simulink library "AVE_Library"  (R2025b)
settings: Solver=VariableStepAuto  StartTime=0.0  StopTime=10.0  RelTol=1e-3
undefined symbols (not defined in the file or in its folder): DiscIntNeverNeededParam
libraries: simulink x44, etargetslib x18, $bdroot x13, GenericTarget x2
(part 1 of 5)
settings Model: Creator=Scythe  LastModifiedBy=damerius
settings SolverCC: AlgebraicLoopSolver=TrustRegion
settings DataIOCC: ReturnWorkspaceOutputs=off
settings OptimizationCC: ReuseModelBlockBuffer=off
settings DebuggingCC: UnconnectedInputMsg=warning  UnconnectedOutputMsg=warning  UnconnectedLineMsg=warning  ArithmeticOperatorsInVariantConditions=warning
settings ModelReferenceCC: EnableRefExpFcnMdlSchedulingChecks=on
settings SFSimCC: CustomCodeUndefinedFunction=UseInterfaceOnly
settings RTWCC: GPUComputeCapability=3.5  DLArmComputeVersion=19.05

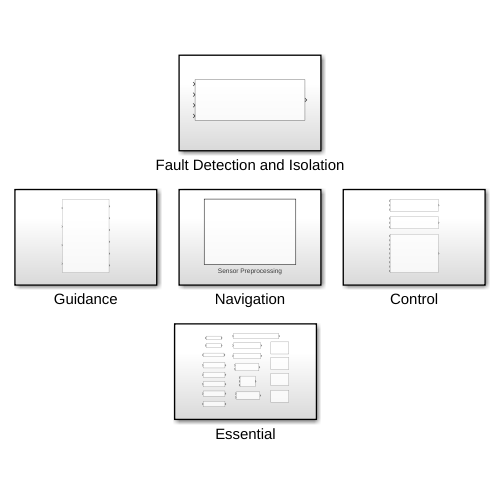
[thumbnail: Simulink's stored preview of the top-level diagram]
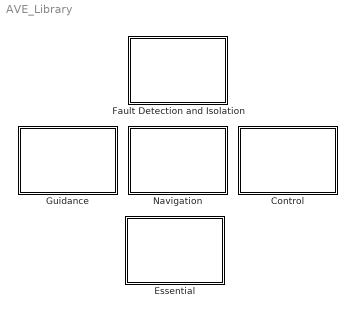
== system AVE_Library ==
  Control : Subsystem
  Essential : Subsystem
  Fault Detection and Isolation : Subsystem
  Guidance : Subsystem
  Navigation : Subsystem

== system AVE_Library/Control ==
  Aperiodic IT2 SISO Control with Integral Action and Input Delay : Subsystem  mask{maxNumDelays=20, SampleTime=0.01}
      mask prompts: maxNumDelays "Max. number of delays:"; SampleTime "Sample time:"
      mask help:
      | Aperiodic SISO controller with integral action for an IT2 process with input delay. The controller is designed online when parameters are changed. The input <b>gamma</b> sets the performance of the controller (<i>mu</i> and <i>beta</i> are optional tuning parameters and can be left to their default values).<br><br>
      | The state-space model being controlled is given by:<br>
      | A = [0 1 0; 0 -1/T1 k/T1; 0 0 -1/T2]<br>
      | B = [0; 0; 1/T2]<br>
      | C = [1 0 0]<br>
      | <br><br>
      | To compensate for input delays, this block stores the previous input values in a ring buffer. The maximum size of the ring buffer is set via the block mask parameter below.
      | <br><br>
      | <table border="1" align="center" width="100%"><tr><th>Input</th></tr></table><br><br>
      | <b>yr_minus_y</b><br>
      | The control error given by the difference of reference value <i>yr</i> and output value <i>y</i>.<br><br>
      | <b>x</b><br>
      | The three-dimensional state vector.<br><br>
      | <table border="1" align="center" width="100%"><tr><th>Input / Parameter</th></tr></table><br><br>
      | <b>k</b>, <b>T1</b>, <b>T2</b><br>Gain and timeconstants of the IT2 process.<br><br>
      | <b>gamma</b> (0,inf)<br>Performance parameter for control design: dominant eigenvalue of closed loop system should be gamma times dominant eigenvalue of model (1/max(T1,T2)). Greater values result in higher performance.<br><br>
      | <b>mu</b> [1, inf)<br>Default value: 2. Spreads 4 poles of closed loop system to the left based on dominant closed loop eigenvalue. A value of 1 means: all poles of closed loop system should be equal to the dominant pole.<br><br>
      | <b>beta</b> [0, inf)<br>Default value: 1. Adjusts the anti-windup gain for back calculation. A value of zero disables back calculation.<br><br>
      | <b>inputTimeDelay</b> [0,inf)<br>Input delay of the process in seconds or zero if the process has no input delay. Internally, this value is rounded to multiples of the sample time and is also clamped to the maximum possible input delay depending on the input ring buffer size.<br><br>
      | <b>saturationLimits</b><br>A two-dimensional vector containing the lower and upper saturation limits. The order does not matter: internally the greatest and lowest value of both are used as upper and lower limit, respectively.<br><br>
      | <b>reset</b><br>Reset the controller by forcing all storage values to zero, including integrator state and the ring buffer for delayed inputs.<br><br>
      | <table border="1" align="center" width="100%"><tr><th>Output</th></tr></table><br><br>
      | <b>u</b><br>The saturated control input to be applied to the process.
      mask DialogControl DescGroupVar Prompt: Aperiodic IT2 SISO Control with Integral Action and Input Delay
      mask Display: disp('Aperiodic IT2 SISO Control\n(Integral Action)\n(Input Delay)');
  Input Delay Compensation : Subsystem  mask{dimU=1, dimX=2, maxNumDelays=20, SampleTime=0.01}
      mask prompts: dimU "Input dimension:"; dimX "State dimension:"; maxNumDelays "Max. number of delays:"; SampleTime "Sample time:"
      mask help:
      | Calculate the input delay compensation term based on the input value of the previous time step and the designed compensation weights. Use this block in conjunction with the "Input Delay Compensation Design" block.<br>
      | This block stores all input values u_prev in a ring buffer and weights all of them by the delayWeights to calculate the compensation term xc. Use the reset input to reset the buffer to zero before storing the input value.<br>
      | <br>
      | <b>Details</b><br>
      | To consider input delays for a linear state space [<i><b>A</b></i>, <i><b>B</b></i>] with control law <i><b>u</b> = -<b>K</b>*<b>x</b></i>, the control law should be replaced by <i><b>u</b> = -<b>Kc</b> * (<b>x</b> + <b>xc</b>)</i>, where <i><b>Kc</b></i> is designed for the state space [<i><b>A</b></i>, <i>expm(-<b>A</b>*h)*<b>B</b></i>] and <i>h &gt; 0</i> is the input delay. <i><b>xc</b></i> is denoted as the compensation term given by the integral of <i>expm(-<b>A</b>*(s+h))*<b>B</b>*u(t+s)</i> over the time interval <i>s=[-h, 0]</i>. For more details, view the reference.
      | <br>
      | <br>
      | <i>Reference<br>
      | Kwon, W. and Pearson, A. (1980). Feedback stabilization of linear systems with delayed control. IEEE Transactions on Automatic Control, 25(2), 266–269. doi:10.1109/TAC.1980.1102288.</i>
      mask DialogControl DescGroupVar Prompt: Input Delay Compensation
      mask Display: disp('Input Delay Compensation');
  Input Delay Compensation Design : Subsystem  mask{dimU=1, dimX=2, maxNumDelays=20, SampleTime=0.01}
      mask prompts: dimU "Input dimension:"; dimX "State dimension:"; maxNumDelays "Max. number of delays:"; SampleTime "Sample time (for design only):"
      mask help:
      | Design weighting matrix for an input delay compensation system. Use this block in conjunction with an "Input Delay Compensation" block. inputDelaySteps represent the input delay in number of discrete time steps with a sampletime specified via the block mask. The sample time parameter is only used to calculate the delay weights. It does not affect the execution of this block.<br>
      | <br>
      | <b>Details</b><br>
      | To consider input delays for a linear state space [<i><b>A</b></i>, <i><b>B</b></i>] with control law <i><b>u</b> = -<b>K</b>*<b>x</b></i>, the control law should be replaced by <i><b>u</b> = -<b>Kc</b> * (<b>x</b> + <b>xc</b>)</i>, where <i><b>Kc</b></i> is designed for the state space [<i><b>A</b></i>, <i>expm(-<b>A</b>*h)*<b>B</b></i>] and <i>h &gt; 0</i> is the input delay. <i><b>xc</b></i> is denoted as the compensation term given by the integral of <i>expm(-<b>A</b>*(s+h))*<b>B</b>*u(t+s)</i> over the time interval <i>s=[-h, 0]</i>. For more details, view the reference.
      | <br>
      | <br>
      | <i>Reference<br>
      | Kwon, W. and Pearson, A. (1980). Feedback stabilization of linear systems with delayed control. IEEE Transactions on Automatic Control, 25(2), 266–269. doi:10.1109/TAC.1980.1102288.</i>
      mask DialogControl DescGroupVar Prompt: Input Delay Compensation Design
      mask Display: disp('Input Delay Compensation\nDesign');

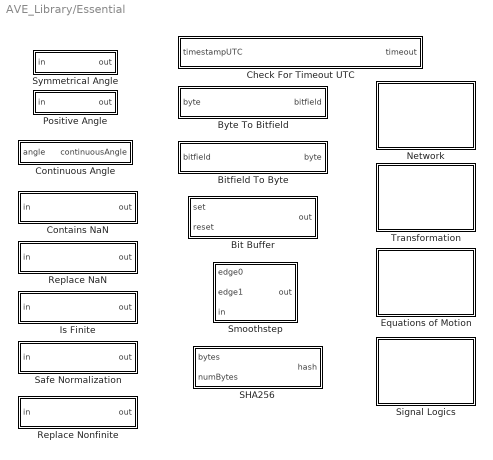
== system AVE_Library/Essential ==
  Bit Buffer : Subsystem  mask{dataType=uint8}
      mask prompts: dataType "Data type:"
      mask help: This block stores all bits in a buffer. All bits from the input "set" are set using bitwise OR of input and buffer. All bits in the buffer remain high until the corresponding bit is reset using the "reset" input. "reset" always overwrites "set".
      mask DialogControl DescGroupVar Prompt: Bit Buffer
      mask Display:
      | type = get_param(gcb, 'dataType');
      | disp(['Bit Buffer\n(' type ')']);
  Bitfield To Byte : Subsystem
      mask help: Convert a bitfield of 8 bits to a single byte. The input bitfield must be a vector containing 8 boolean values where the first value indicates whether the LSBit is to be set or not.
      mask DialogControl DescGroupVar Prompt: Bitfield To Byte
      mask Display: text(0.5, 0.5, 'Bitfield to Byte', 'horizontalAlignment', 'center');
  Byte To Bitfield : Subsystem
      mask help: Extract all bits from a single byte. The bitfield output contains 8 boolean values where the first value indicates whether the LSBit is set or not.
      mask DialogControl DescGroupVar Prompt: Byte To Bitfield
      mask Display: text(0.5, 0.5, 'Byte to Bitfield', 'horizontalAlignment', 'center');
  Check For Timeout UTC : Subsystem  mask{timeout=1, sampleTime=-1}
      mask prompts: timeout "Timeout in seconds:"; sampleTime "Sampletime (-1 for inherited):"
      mask help:
      | Check for timeout by detecting the progress of a UTC timestamp signal. The UTC timestamp signal must move on within the specified timeout value, otherwise the output is set to true. The output signal is true as long as the timeout is present.<br><br>
      | <i><b>Note:</b> This block requires the GenericTarget Toolbox to be installed!</i>
      mask DialogControl DescGroupVar Prompt: Check For Timeout UTC
      mask Display:
      | maskStr = get_param(gcb,'timeout');
      | strText = ['Check For Timeout UTC\n(' maskStr ' s)'];
      | disp(strText);
  Contains NaN : Subsystem
      mask help: Outputs true if any value in the input contains NaN values.
      mask DialogControl DescGroupVar Prompt: Contains NaN
      mask Display: disp('Contains NaN')
  Continuous Angle : Subsystem
      mask help: Convert a given angle [rad] to a continuous output angle [rad]. The difference of the current angle input to the previous angle input is used to update an internal integrator.
      mask DialogControl DescGroupVar Prompt: Continuous Angle
  Equations of Motion : Subsystem
  Is Finite : Subsystem
      mask help: Check whether the input is finite or not. The input must be of type 'double'. The output is of type 'boolean' and has the same dimension as the input. An element in the output is true, if the corresponding element of the input is finite.
      mask DialogControl DescGroupVar Prompt: Is Finite
      mask Display: disp('Is Finite');
  Network : Subsystem
  Positive Angle : Subsystem
      mask help: Convert a given angle [rad] to an output angle [rad] with the output angle being in range [0, +2*pi).
      mask DialogControl DescGroupVar Prompt: Positive Angle
      mask Display:
      | % Get dimension of block
      | pos = get_param(gcb, 'Position');
      | width = pos(3) - pos(1);
      | height = pos(4) - pos(2);
      | 
      | % Set equation
      | text(0.5*width,0.5*height,'[0, +2\pi)', 'hor','center','texmode','on');
  Replace NaN : Subsystem  mask{value=0.0}
      mask prompts: value "Replace NaN by:"
      mask help: Assign the input to the output but replace all NaN values from the input by a specified value.
      mask DialogControl DescGroupVar Prompt: Replace NaN
      mask Display:
      | maskStr = get_param(gcb,'value');
      | disp(['Replace NaN\n(',maskStr,')']);
  Replace Nonfinite : Subsystem  mask{value=0}
      mask prompts: value "Replace Nonfinite by:"
      mask help: Assign the input to the output but replace all nonfinite values from the input by a specified value.
      mask DialogControl DescGroupVar Prompt: Replace Nonfinite
      mask Display:
      | maskStr = get_param(gcb,'value');
      | disp(['Replace Nonfinite\n(',maskStr,')']);
  SHA256 : Subsystem
      mask help: Calculate the 256-bit hash (SHA256) for given binary data.
      mask DialogControl DescGroupVar Prompt: SHA256
      mask Display: disp('SHA256');
  Safe Normalization : Subsystem
      mask help: Normalize the input vector. The resulting output vector is ensured to have unit length. If the input contains non-finite values or represents a zero-length vector, then a default output vector is generated, where the first element is one and all remaining elements are zero.
      mask DialogControl DescGroupVar Prompt: Safe Normalization
      mask Display: disp('Safe\nNormalization');
  Signal Logics : Subsystem
  Smoothstep : Subsystem
      mask help:
      | A smooth interpolation function between two values [edge0, edge1] with f(edge0)=0, f(edge1)=1.<br><br>
      |
      | <b>edge0</b><br>Edge value where the output should be zero.<br><br>
      | <b>edge1</b><br>Edge value where the output should be one.<br><br>
      | <b>in</b><br>Function value where to calculate the interpolation value.
      mask DialogControl DescGroupVar Prompt: Smoothstep
      mask Display:
      | % Get dimension of block
      | pos = get_param(gcb, 'Position');
      | width = pos(3) - pos(1);
      | height = pos(4) - pos(2);
      | 
      | % Set image to center of block
      | image('AVE_Icon_Smoothstep.svg');
  Symmetrical Angle : Subsystem
      mask help: Convert a given angle [rad] to an output angle [rad] with the output angle being in range [-pi, +pi).
      mask DialogControl DescGroupVar Prompt: Symmetrical Angle
      mask Display:
      | % Get dimension of block
      | pos = get_param(gcb, 'Position');
      | width = pos(3) - pos(1);
      | height = pos(4) - pos(2);
      | 
      | % Set equation
      | text(0.5*width,0.5*height,'[-\pi, +\pi)', 'hor','center','texmode','on');
  Transformation : Subsystem

== system AVE_Library/Fault Detection and Isolation ==
  Robust Deviation Detection : Subsystem
      mask help:
      | Detect a deviation in the residual signal. The residual signal should be normal distributed with zero mean in the fault free case. Deviations of at least [minDetectableDeviation] are detected within maximum  [maxNumSamplesForDetection]. You should enter your maximum tollerable values to avoid false alarms.<br><br>
      |
      | <table border="1" align="center" width="100%"><tr><th>Input</th></tr></table><br><br>
      | <b>timestamp</b><br>
      | N-by-1 vector indicating the timestamp of the corresponding measurement. A change of the timestamp indicates a new measurement.<br><br>
      |
      | <b>residualSignal</b><br>
      | N-by-1 vector containing N measurements representing a residual signal. This can be the difference between an expected value and a measured value.  The corresponding timestamp of a residual signal is given by the timestamp input.<br><br>
      |
      | <b>minDetectableDeviation</b><br>
      | The deviation from zero that is guaranteed to be detected within the given number of samples.
      | The fault free signal is defined to be mostly between  +-(minDetectableDeviation)*2/3.<br><br>
      |
      | <b>maxNumSamplesForDetection</b><br>
      | The time in samples used in maximum for detection of fault. (nSamples max tolerable detection delay) = (max DetectionTime seconds) / Sampletime<br><br>
      |
      | <table border="1" align="center" width="100%"><tr><th>Output</th></tr></table><br><br>
      |
      | <b>faultIsActive</b><br>
      | N-by-1 vector indicating whether a fault is active (true) or not (false) with N being the number of input measurements<br><br>
      |
      | <b>faultDetectionTime</b><br>
      | Time, when fault is detected, which is later than fault occurence time.<br><br>
      |
      | <b>faultOccurenceTime</b><br>
      | Time, when fault has occured, which is detected later at faultDetectionTime.<br><br>
      |
      | <b>faultCounter</b><br>
      | counts +one when faultActive switches from false to true.<br><br>
      |
      | <b>faultClearedDetectionTime</b><br>
      | Time at which it is detected that the fault has disappeared.<br><br>
      |
      | <b>estimatedFaultClearedTime</b><br>
      | Time at which a fault has disappeared.<br><br>
      |
      | <b>worstSiturationTime</b><br>
      | Even if no fault has occurred, this value represents the time of the maximum worst situation which is not always the maximum deviation when it is just for a very short time.<br><br>
      |
      | <b>decisionFunctionDiagnostics</b><br>
      | The debug signal "decisionFunctionDiagnostic" can be used to check how close the evaluation is to an alarm/false alarm. The signal shown increases with probability of an alarm and moves towards zero if there is no error. As soon as the drawn threshold is exceeded, an error detection is triggered.<br><br>
      mask DialogControl DescGroupVar Prompt: Robust Deviation Detection
      mask Display: disp('Robust\nDeviation Detection');

== system AVE_Library/Guidance ==
  Trajectory Track Error : Subsystem
      mask help:
      | Calculate the track error to a given trajectory and get the indices and interpolation value for the closest point and the target point. All input positions are transformed to an euclidian NED frame. Therefore, this function may not be used if the points of the trajectory are too far apart.<br><br>
      | <table border="1" align="center" width="100%"><tr><th>Input</th></tr></table><br><br>
      |
      | <b>time</b><br>
      | The current time value to be compared with the trajectory. If the time is not within the range of the trajectory time window, then the valid output remains false (invalid).<br><br>
      |
      | <b>positionLLA</b><br>The geographic position of the vehicle for which to calculate the distance to the trajectory. The elements are<br>
      | 1: latitude (radians)<br>
      | 2: longitude (radians)<br>
      | 3: altitude (meters, positive upwards)<br><br>
      |
      | <b>matTimeLatLon</b><br>
      | N-by-3 matrix representing the time and 2D geographic position data of the trajectory. Each row indicates one point of the trajectory. The format of one row is as follows:<br>
      | 1: time (seconds), must be monotonically increasing<br>
      | 2: latitude (radians)<br>
      | 3: longitude (radians)<br><br>
      |
      | <b>numPoints</b><br>
      | The actual number of columns from the matTimeLatLon matrix to be considered for the calculation.<br><br>
      |
      | <table border="1" align="center" width="100%"><tr><th>Output</th></tr></table><br><br>
      |
      | <b>valid</b><br>
      | True if all outputs are valid and the computation was successful, false otherwise. The output is invalid, if the input time is not within the time range of the trajectory, if the number of points is less than 2 or some numerical problems occured (e.g. two points were to close to compute a line).<br><br>
      |
      | <b>trackError</b><br>
      | 2-dimensional vector containing track errors xb (along the track) and yb (cross track error). The elements are as follows<br>
      | 1: xb, error from the closest point to the trajectory to the target point of the trajectory (according to given input time). This value is an accumulation of all line segments in between. xb is positive if the target point is "after" the closest point.<br>
      | 2: yb, lateral distance to the closest line segment of the trajectory. yb is positive if the vehicle is "on the right" of the trajectory.<br>
      | If the vehicle is "before" or "after" the trajectory, then an extrapolated point according to the first or last line segment is calculated. xb and yb then take the distance to this extrapolated line into account.<br><br>
      |
      | <b>closestSegmentIndices</b><br>
      | The two indices of the line segment that is closest to the vehicle position. If the output is not valid, these values are undefined.<br><br>
      |
      | <b>closestSegmentLinearInterpolationRatio</b><br>
      | The scalar interpolation ratio for the closest line segment. The indices of the line segment indicate two values v1 and v2. The interpolated value is calculated by v = v1 + ratio*(v2 - v1).<br><br>
      |
      | <b>targetSegmentIndices</b><br>
      | The two indices of the line segment that contain the target position (according to the input time). If the output is not valid, these values are undefined.<br><br>
      |
      | <b>targetSegmentLinearInterpolationRatio</b><br>
      | The scalar interpolation ratio for the target line segment. The indices of the line segment indicate two values v1 and v2. The interpolated value is calculated by v = v1 + ratio*(v2 - v1).<br><br>
      mask DialogControl DescGroupVar Prompt: Trajectory Track Error
      mask Display: disp('Trajectory\nTrack Error');

== system AVE_Library/Navigation ==
  Sensor Preprocessing : Subsystem

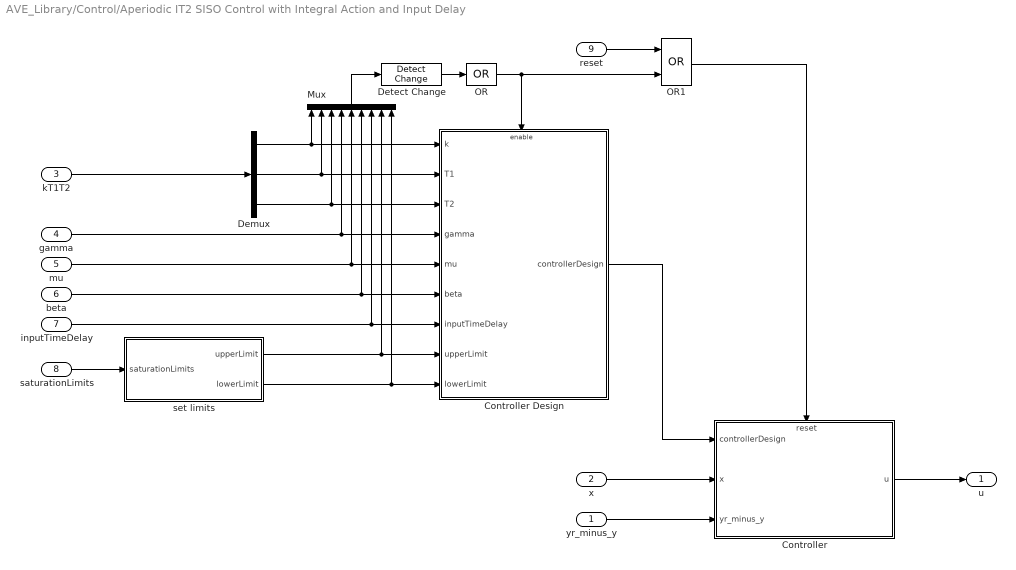
== system AVE_Library/Control/Aperiodic IT2 SISO Control with Integral Action and Input Delay ==
  yr_minus_y : Inport  OutDataTypeStr=double  PortDimensions=1  SampleTime=SampleTime
  x : Inport  Port=2  OutDataTypeStr=double  PortDimensions=3  SampleTime=SampleTime
  kT1T2 : Inport  Port=3  OutDataTypeStr=double  PortDimensions=3
  gamma : Inport  Port=4  OutDataTypeStr=double  PortDimensions=1
  mu : Inport  Port=5  OutDataTypeStr=double  PortDimensions=1
  beta : Inport  Port=6  OutDataTypeStr=double  PortDimensions=1
  inputTimeDelay : Inport  Port=7  OutDataTypeStr=double  Unit=s  PortDimensions=1
  saturationLimits : Inport  Port=8
  reset : Inport  Port=9  OutDataTypeStr=boolean  PortDimensions=1  SampleTime=SampleTime
  Controller : Subsystem
      settings: PortSchema="{\"entries\":[{\"content\":{\"sides\":[{\"content\":{\"connectorIds\":[\"In1\",\"In2\",\"In3\"]},\"type\":\"ConnectorPlacement.EquallySpacedRectSide\",\"uuid\":\"2441c3d9-9036-4959-8654-38bcf7512db1\"},{\"content\":{\"connectorIds\":[\"Out1\"],\"side\":\"RIGHT\"},\"type\":\"ConnectorPlacement.EquallySpacedRectSide\",\"uuid\":\"09d94185-6b81-4a2e-aa7e-c9238ca87f8c\"},{\"content\":{\"connectorIds\":[\"In4\"],\"side\":\"TOP\"},\"type\":\"ConnectorPlacement.EquallySpacedRectSide\",\"uuid\":\"d5fce340-7cee-4420-ba63-1b0e5fdd6ba2\"}]},\"type\":\"ConnectorPlacement.EquallySpacedConnector\",\"uuid\":\"db3004f6-d6ef-47ec-b025-84b5b26d9b06\"}],\"packageUris\":[\"http://schema.mathworks.com/mf0/Connector/R2020b\"],\"version\":\"1.0\"}"
  Controller Design : Subsystem
  Demux : Demux  Outputs=3
  Detect Change : simulink/Logic and Bit Operations/Detect Change  vinit=0  OutDataTypeStr=boolean
  Mux : Mux  Inputs=9
  OR : Logic  Operator=OR  Inputs=1  AllPortsSameDT=off  OutDataTypeStr=boolean
  OR1 : Logic  Operator=OR  AllPortsSameDT=off  OutDataTypeStr=boolean
  set limits : Subsystem
  u : Outport  OutDataTypeStr=double  PortDimensions=1  SampleTime=SampleTime
  wires:
  OR1/1 -> Controller/4(reset)
  OR/1 -> Controller Design/Enable, OR1/2
  Detect Change/1 -> OR/1
  Mux/1 -> Detect Change/1
  Controller/1(u) -> u/1
  set limits/2(lowerLimit) -> Controller Design/9(lowerLimit), Mux/9
  set limits/1(upperLimit) -> Controller Design/8(upperLimit), Mux/8
  reset/1 -> OR1/1
  Controller Design/1(controllerDesign) -> Controller/1(controllerDesign)
  yr_minus_y/1 -> Controller/3(yr_minus_y)
  x/1 -> Controller/2(x)
  beta/1 -> Controller Design/6(beta), Mux/6
  mu/1 -> Controller Design/5(mu), Mux/5
  Demux/2 -> Controller Design/2(T1), Mux/2
  Demux/3 -> Controller Design/3(T2), Mux/3
  gamma/1 -> Controller Design/4(gamma), Mux/4
  Demux/1 -> Controller Design/1(k), Mux/1
  inputTimeDelay/1 -> Controller Design/7(inputTimeDelay), Mux/7
  kT1T2/1 -> Demux/1
  saturationLimits/1 -> set limits/1(saturationLimits)

== system AVE_Library/Control/Input Delay Compensation ==
  u_prev : Inport  OutDataTypeStr=double  PortDimensions=dimU  SampleTime=SampleTime
  delayWeights : Inport  Port=2  OutDataTypeStr=double  PortDimensions=[dimX, dimU*maxNumDelays]  SampleTime=SampleTime
  reset : Inport  Port=3  OutDataTypeStr=boolean  PortDimensions=1  SampleTime=SampleTime
  Calculate Compensation Term : MATLAB Function  TreatAsAtomicUnit=on
  Reshape : Reshape  OutputDimensionality=Column vector (2-D)
  xc : Outport  OutDataTypeStr=double  PortDimensions=dimX  SampleTime=SampleTime
  wires:
  u_prev/1 -> Reshape/1
  Calculate Compensation Term/1(x) -> xc/1
  Reshape/1 -> Calculate Compensation Term/1(u_prev)
  delayWeights/1 -> Calculate Compensation Term/2(weightMatrixStack)
  reset/1 -> Calculate Compensation Term/3(reset)

== system AVE_Library/Control/Input Delay Compensation Design ==
  A : Inport  OutDataTypeStr=double  PortDimensions=[dimX, dimX]
  B : Inport  Port=2  OutDataTypeStr=double  PortDimensions=[dimX, dimU]
  inputDelaySteps : Inport  Port=3  OutDataTypeStr=int32  PortDimensions=1
  calculate weight matrix stack : MATLAB Function  TreatAsAtomicUnit=on
  delayWeights : Outport  OutDataTypeStr=double  PortDimensions=[dimX, dimU*maxNumDelays]
  wires:
  inputDelaySteps/1 -> calculate weight matrix stack/3(num_delay_steps)
  A/1 -> calculate weight matrix stack/1(A)
  B/1 -> calculate weight matrix stack/2(B)
  calculate weight matrix stack/1(W) -> delayWeights/1

== system AVE_Library/Essential/Bit Buffer ==
  set : Inport  OutDataTypeStr=dataType  PortDimensions=1
  reset : Inport  Port=2  OutDataTypeStr=dataType
  BitwiseAND : simulink/Logic and Bit Operations/Bitwise Operator  logicop=AND  UseBitMask=off  NumInputPorts=2  BitMask=bin2dec('11011001')  BitMaskRealWorld=Stored Integer
  BitwiseNOT : simulink/Logic and Bit Operations/Bitwise Operator  logicop=NOT  UseBitMask=off  BitMask=bin2dec('11011001')  BitMaskRealWorld=Stored Integer
  BitwiseOR : simulink/Logic and Bit Operations/Bitwise Operator  logicop=OR  UseBitMask=off  NumInputPorts=2  BitMask=bin2dec('11011001')  BitMaskRealWorld=Stored Integer
  Unit Delay1 : UnitDelay  SampleTime=-1  HasFrameUpgradeWarning=on
  out : Outport  OutDataTypeStr=dataType
  wires:
  set/1 -> BitwiseOR/1
  Unit Delay1/1 -> BitwiseOR/2
  BitwiseNOT/1 -> BitwiseAND/1
  BitwiseAND/1 -> Unit Delay1/1, out/1
  reset/1 -> BitwiseNOT/1
  BitwiseOR/1 -> BitwiseAND/2

== system AVE_Library/Essential/Bitfield To Byte ==
  bitfield : Inport  OutDataTypeStr=boolean  PortDimensions=8
  Bitwise Operator : simulink/Logic and Bit Operations/Bitwise Operator  logicop=OR  UseBitMask=off  NumInputPorts=8  BitMask=bin2dec('11011001')  BitMaskRealWorld=Stored Integer
  Data Type Conversion : DataTypeConversion  OutDataTypeStr=uint8  SaturateOnIntegerOverflow=off  RndMeth=Floor
  Demux : Demux  Outputs=8
  Shift Arithmetic : ArithShift  BitShiftNumber=1  BitShiftDirection=Left
  Shift Arithmetic1 : ArithShift  BitShiftNumber=2  BitShiftDirection=Left
  Shift Arithmetic2 : ArithShift  BitShiftNumber=3  BitShiftDirection=Left
  Shift Arithmetic3 : ArithShift  BitShiftNumber=4  BitShiftDirection=Left
  Shift Arithmetic4 : ArithShift  BitShiftNumber=5  BitShiftDirection=Left
  Shift Arithmetic5 : ArithShift  BitShiftNumber=6  BitShiftDirection=Left
  Shift Arithmetic6 : ArithShift  BitShiftNumber=7  BitShiftDirection=Left
  byte : Outport  OutDataTypeStr=uint8  PortDimensions=1
  wires:
  bitfield/1 -> Data Type Conversion/1
  Shift Arithmetic6/1 -> Bitwise Operator/8
  Shift Arithmetic2/1 -> Bitwise Operator/4
  Bitwise Operator/1 -> byte/1
  Shift Arithmetic3/1 -> Bitwise Operator/5
  Shift Arithmetic4/1 -> Bitwise Operator/6
  Demux/8 -> Shift Arithmetic6/1
  Demux/5 -> Shift Arithmetic3/1
  Demux/3 -> Shift Arithmetic1/1
  Demux/2 -> Shift Arithmetic/1
  Demux/6 -> Shift Arithmetic4/1
  Shift Arithmetic1/1 -> Bitwise Operator/3
  Demux/1 -> Bitwise Operator/1
  Shift Arithmetic5/1 -> Bitwise Operator/7
  Demux/7 -> Shift Arithmetic5/1
  Shift Arithmetic/1 -> Bitwise Operator/2
  Data Type Conversion/1 -> Demux/1
  Demux/4 -> Shift Arithmetic2/1

== system AVE_Library/Essential/Byte To Bitfield ==
  byte : Inport  OutDataTypeStr=uint8  PortDimensions=1
  Bitwise Operator : simulink/Logic and Bit Operations/Bitwise Operator  logicop=AND  UseBitMask=on  BitMask=1  BitMaskRealWorld=Stored Integer
  Bitwise Operator1 : simulink/Logic and Bit Operations/Bitwise Operator  logicop=AND  UseBitMask=on  BitMask=2  BitMaskRealWorld=Stored Integer
  Bitwise Operator2 : simulink/Logic and Bit Operations/Bitwise Operator  logicop=AND  UseBitMask=on  BitMask=4  BitMaskRealWorld=Stored Integer
  Bitwise Operator3 : simulink/Logic and Bit Operations/Bitwise Operator  logicop=AND  UseBitMask=on  BitMask=8  BitMaskRealWorld=Stored Integer
  Bitwise Operator4 : simulink/Logic and Bit Operations/Bitwise Operator  logicop=AND  UseBitMask=on  BitMask=16  BitMaskRealWorld=Stored Integer
  Bitwise Operator5 : simulink/Logic and Bit Operations/Bitwise Operator  logicop=AND  UseBitMask=on  BitMask=32  BitMaskRealWorld=Stored Integer
  Bitwise Operator6 : simulink/Logic and Bit Operations/Bitwise Operator  logicop=AND  UseBitMask=on  BitMask=64  BitMaskRealWorld=Stored Integer
  Bitwise Operator7 : simulink/Logic and Bit Operations/Bitwise Operator  logicop=AND  UseBitMask=on  BitMask=128  BitMaskRealWorld=Stored Integer
  Data Type Conversion1 : DataTypeConversion  OutDataTypeStr=boolean  SaturateOnIntegerOverflow=off  RndMeth=Floor
  Mux : Mux  Inputs=8
  bitfield : Outport  OutDataTypeStr=boolean  PortDimensions=8
  wires:
  Mux/1 -> Data Type Conversion1/1
  byte/1 -> Bitwise Operator1/1, Bitwise Operator2/1, Bitwise Operator3/1, Bitwise Operator4/1, Bitwise Operator5/1, Bitwise Operator6/1, Bitwise Operator7/1, Bitwise Operator/1
  Bitwise Operator/1 -> Mux/1
  Bitwise Operator1/1 -> Mux/2
  Bitwise Operator2/1 -> Mux/3
  Bitwise Operator3/1 -> Mux/4
  Bitwise Operator4/1 -> Mux/5
  Bitwise Operator5/1 -> Mux/6
  Bitwise Operator6/1 -> Mux/7
  Bitwise Operator7/1 -> Mux/8
  Data Type Conversion1/1 -> bitfield/1

== system AVE_Library/Essential/Check For Timeout UTC ==
  timestampUTC : Inport  OutDataTypeStr=double  Unit=s  PortDimensions=1
  Compare To Constant : simulink/Logic and Bit Operations/Compare To Constant  relop=>=  const=timeout  OutDataTypeStr=boolean
  Enabled Subsystem : Subsystem  TreatAsAtomicUnit=on
  Model Execution Time : GenericTarget/Time/Model Execution Time  SampleTime=sampleTime
      settings: SourceProductName=Generic Target
  Sum : Sum  Inputs=|-+
  UTC Timestamp Moved On : GenericTarget/Time/UTC Timestamp Moved On  vinit=0
      settings: SourceProductName=Generic Target
  timeout : Outport  OutDataTypeStr=boolean  PortDimensions=1
  wires:
  Compare To Constant/1 -> timeout/1
  timestampUTC/1 -> UTC Timestamp Moved On/1
  Sum/1 -> Compare To Constant/1
  Model Execution Time/1 -> Enabled Subsystem/1(In1), Sum/2
  UTC Timestamp Moved On/1 -> Enabled Subsystem/Enable
  Enabled Subsystem/1(Out1) -> Sum/1

== system AVE_Library/Essential/Contains NaN ==
  in : Inport
  MATLAB Function : MATLAB Function  TreatAsAtomicUnit=on
  out : Outport  OutDataTypeStr=boolean  PortDimensions=1
  wires:
  in/1 -> MATLAB Function/1(u)
  MATLAB Function/1(y) -> out/1

== system AVE_Library/Essential/Continuous Angle ==
  angle : Inport  OutDataTypeStr=double  Unit=rad
  Add : Sum
  Add2 : Sum  Inputs=+-
  Ensure Symmetrical Input : $bdroot/Essential/Symmetrical Angle
  Memory1 : Memory
  Output Buffer : Memory
  Symmetrical Angle : $bdroot/Essential/Symmetrical Angle
  continuousAngle : Outport  OutDataTypeStr=double  Unit=rad
  wires:
  Add/1 -> continuousAngle/1, Output Buffer/1
  Ensure Symmetrical Input/1 -> Add2/1, Memory1/1
  Memory1/1 -> Add2/2
  Output Buffer/1 -> Add/2
  Symmetrical Angle/1 -> Add/1
  Add2/1 -> Symmetrical Angle/1
  angle/1 -> Ensure Symmetrical Input/1

== system AVE_Library/Essential/Equations of Motion ==
  Kinematic 3DoF Euclidean : Subsystem
      mask help:
      | Continuous kinematic simulation in 3 degrees of freedom (DoF) for euclidean motion.<br><br>
      |
      | <br><table border="1" align="center" width="100%"><tr><th>Input</th></tr></table><br><br>
      | <b>uvr</b><br>
      | 3-dimensional vector, representing the translational velocity (uv) and rotational velocity (r) of the body-frame with respect to the navigation-frame in coordinates of the body-frame.
      | <br><br>
      |
      | <b>initialPoseXYPsi</b><br>
      | 3-dimensional vector representing the initial euclidean pose (x [m], y[m] and psi [rad]).
      | <br><br>
      |
      | <b>reset</b><br>
      | True if internal state should be reset to the specified initial values.
      | <br><br>
      |
      | <br><table border="1" align="center" width="100%"><tr><th>Output</th></tr></table><br><br>
      | <b>poseXYPsi</b><br>
      | 3-dimensional vector representing the resulting euclidean pose (x [m], y[m] and psi [rad]).
      mask DialogControl DescGroupVar Prompt: Kinematic 3DoF Euclidean
      mask Display: disp('Kinematic 3DoF\n(Euclidean)');
  Kinematic 6DoF Geographic : Subsystem
      mask help:
      | Continuous kinematic simulation in 6 degrees of freedom (DoF) for geographic (WGS84) motion.<br><br>
      |
      | <br><table border="1" align="center" width="100%"><tr><th>Input</th></tr></table><br><br>
      | <b>uvwpqr</b><br>
      | 6-dimensional vector, representing the translational velocity (uvw) and rotational velocity (pqr) of the body-frame with respect to the navigation-frame in coordinates of the body-frame.
      | <br><br>
      |
      | <b>initialLatLonAlt</b><br>
      | 3-dimensional vector representing the initial geographic position (latitude [rad], longitude [rad] and altitude [m]).
      | <br><br>
      |
      | <b>initialRollPitchYaw</b><br>
      | 3-dimensional vector representing the initial orientation (roll [rad], pitch [rad] and yaw [rad]).
      | <br><br>
      |
      | <b>reset</b><br>
      | True if internal state should be reset to the specified initial values.
      | <br><br>
      |
      | <br><table border="1" align="center" width="100%"><tr><th>Output</th></tr></table><br><br>
      | <b>busState</b><br>
      | A bus representing the motion state. The positionNED denotes the euclidean position with respect to the initial geographic position. The acceleration includes gravity. All velocities denote velocities of the b-frame with respect to the n-frame given in either b-frame or n-frame coordinates. The state bus contains the following elements:<br>
      | <table border="1" cellpadding="5">
      | <tr style="background-color: #D1CBC5;"><th align="left">Name</th><th align="left">Description</th></tr>
      | <tr><td>positionLatitude</td><td>Latitude according to WGS84.</td></tr>
      | <tr><td>positionLongitude</td><td>Longitude according to WGS84.</td></tr>
      | <tr><td>positionAltitude</td><td>Altitude, positive upwards, according to WGS84.</td></tr>
      | <tr><td>positionNorth</td><td>Euclidean position in north direction w.r.t. initialLatLonAlt.</td></tr>
      | <tr><td>positionEast</td><td>Euclidean position in east direction w.r.t. initialLatLonAlt.</td></tr>
      | <tr><td>positionDown</td><td>Euclidean position in down direction w.r.t. initialLatLonAlt.</td></tr>
      | <tr><td>orientationQuaternionW</td><td>Scalar part for the unit quaternion that describes the rotation from body to n-frame.</td></tr>
      | <tr><td>orientationQuaternionX</td><td>X component of the vector part for the unit quaternion that describes the rotation from body to n-frame.</td></tr>
      | <tr><td>orientationQuaternionY</td><td>Y component of the vector part for the unit quaternion that describes the rotation from body to n-frame.</td></tr>
      | <tr><td>orientationQuaternionZ</td><td>Z component of the vector part for the unit quaternion that describes the rotation from body to n-frame.</td></tr>
      | <tr><td>orientationRoll</td><td>Roll angle (euler angle around X axis) in radians according to the ZYX-convention.</td></tr>
      | <tr><td>orientationPitch</td><td>Pitch angle (euler angle around Y axis) in radians according to the ZYX-convention.</td></tr>
      | <tr><td>orientationYaw</td><td>Yaw angle (euler angle around Z axis) in radians according to the ZYX-convention.</td></tr>
      | <tr><td>velocityNorth</td><td>Velocity in north direction.</td></tr>
      | <tr><td>velocityEast</td><td>Velocity in east direction.</td></tr>
      | <tr><td>velocityDown</td><td>Velocity in down direction.</td></tr>
      | <tr><td>velocityU</td><td>Velocity in X direction of the b-frame.</td></tr>
      | <tr><td>velocityV</td><td>Velocity in Y direction of the b-frame.</td></tr>
      | <tr><td>velocityW</td><td>Velocity in Z direction of the b-frame.</td></tr>
      | <tr><td>velocityP</td><td>Rotational velocity of the b-frame w.r.t. n-frame around X axis of the b-frame.</td></tr>
      | <tr><td>velocityQ</td><td>Rotational velocity of the b-frame w.r.t. n-frame around Y axis of the b-frame.</td></tr>
      | <tr><td>velocityR</td><td>Rotational velocity of the b-frame w.r.t. n-frame around Z axis of the b-frame.</td></tr>
      | <tr><td>accelerationNorth</td><td>Acceleration (including gravity) in north direction.</td></tr>
      | <tr><td>accelerationEast</td><td>Acceleration (including gravity) in east direction.</td></tr>
      | <tr><td>accelerationDown</td><td>Acceleration (including gravity) in down direction.</td></tr>
      | <tr><td>accelerationX</td><td>Acceleration (including gravity) in X direction of the b-frame.</td></tr>
      | <tr><td>accelerationY</td><td>Acceleration (including gravity) in Y direction of the b-frame.</td></tr>
      | <tr><td>accelerationZ</td><td>Acceleration (including gravity) in Z direction of the b-frame.</td></tr>
      | <tr><td>courseOverGround</td><td>Course over ground.</td></tr>
      | <tr><td>speedOverGround</td><td>Speed over ground.</td></tr>
      | <tr><td>angleOfAttack</td><td>The angle of attack is defined to be atan2(velocityDown, speedOverGround).</td></tr>
      | <tr><td>sideSlipAngle</td><td>The side slip angle is defined to be (courseOverGround - orientationYaw).</td></tr>
      | <tr><td>pqr_ib</td><td>3-dimensional vector of rotational velocities of the b-frame with respect to an inertial i-frame given in coordinates of the b-frame. This rotational velocity includes the earth rotation and the transport rate due to movement on the ellipsoid. This value corresponds to a a value an inertial measurement unit would measure.</td></tr>
      | </table>
      | <br><br>
      mask DialogControl DescGroupVar Prompt: Kinematic 6DoF Geographic
      mask Display: disp('Kinematic 6DoF\n(Geographic)');
  Strapdown Algorithm : Subsystem
      mask help:
      | Calculate one discrete integration step of the strapdown algorithm. The explicit euler method is used as integration method.<br><br>
      |
      | <br><table border="1" align="center" width="100%"><tr><th>Input</th></tr></table><br><br>
      | <b>sampletime</b><br>
      | Sampletime to be used for integration. Unit is (s).<br><br>
      |
      | <b>imuAcceleration</b><br>
      | Raw acceleration of the IMU. The acceleration bias may be removed. Unit is (m/s^2).<br><br>
      |
      | <b>imuAngularRate</b><br>
      | Raw angular rate of the IMU. The angular rate bias may be removed. Unit is (rad/s).<br><br>
      |
      | <b>positionLLA</b><br>
      | Initial geographic position (latitude [rad], longitude [rad], altitude [m]). The altitude is counted positive upwards.<br><br>
      |
      | <b>orientationQuaternionWXYZ</b><br>
      | Initial unit quaternion representing the orientation of the b-frame with respect to the n-frame. The format is [w;x;y;z], where w denotes the scalar part and [x;y;z] denotes the vector part of the quaternion, respectively.<br><br>
      |
      | <b>velocityUVW</b><br>
      | Initial body-fixed velocity. Unit is (m/s).<br><br>
      |
      | <br><table border="1" align="center" width="100%"><tr><th>Output</th></tr></table><br><br>
      | <b>outPositionLLA</b><br>
      | Output geographic position. The format is equal to the positionLLA input.<br><br>
      |
      | <b>outOrientationQuaternionWXYZ</b><br>
      | Output quaternion. The format is equal to the orientationQuaternionWXYZ input.<br><br>
      |
      | <b>outVelocityUVW</b><br>
      | Output velocity. The format is equal to the velocityUVW input.<br><br>
      mask DialogControl DescGroupVar Prompt: Strapdown Algorithm
      mask Display: disp('Strapdown Algorithm\nOne Step Euler Integration')

== system AVE_Library/Essential/Is Finite ==
  in : Inport  OutDataTypeStr=double
  MATLAB Function : MATLAB Function  TreatAsAtomicUnit=on
  out : Outport  OutDataTypeStr=boolean
  wires:
  MATLAB Function/1(y) -> out/1
  in/1 -> MATLAB Function/1(u)

== system AVE_Library/Essential/Network ==
  Compare IP : Subsystem
      mask help: Compare two IP addresses and return true if both IPv4 addresses are equal. Both inputs are 4-by-1 vectors of type uint8.
      mask DialogControl DescGroupVar Prompt: Compare IP
      mask Display: disp('Compare IP');
  Message MUX : Subsystem
      mask help: MUX two binary messages to one message. The dimension of the output is equal to the sum of the input sizes.
      mask DialogControl DescGroupVar Prompt: Message MUX
      mask Display: disp('Message MUX');
  Swap Double Host To Network : Subsystem
      mask help: Swap bytes of a double value from host byte-order to network byte-order (big-endian).
      mask DialogControl DescGroupVar Prompt: Swap Double Host To Network
      mask Display: disp('hton (double)');
  Swap Float Host To Network : Subsystem
      mask help: Swap bytes of a float value from host byte-order to network byte-order (big-endian).
      mask DialogControl DescGroupVar Prompt: Swap Float Host To Network
      mask Display: disp('hton (float)');
  Swap Int16 Host To Network : Subsystem
      mask help: Swap bytes of an int16 value from host byte-order to network byte-order (big-endian).
      mask DialogControl DescGroupVar Prompt: Swap Int16 Host To Network
      mask Display: disp('hton (int16)');
  Swap Int32 Host To Network : Subsystem
      mask help: Swap bytes of an int32 value from host byte-order to network byte-order (big-endian).
      mask DialogControl DescGroupVar Prompt: Swap Int32 Host To Network
      mask Display: disp('hton (int32)');
  Swap Uint16 Host To Network : Subsystem
      mask help: Swap bytes of a uint16 value from host byte-order to network byte-order (big-endian).
      mask DialogControl DescGroupVar Prompt: Swap Uint16 Host To Network
      mask Display: disp('hton (uint16)');
  Swap Uint32 Host To Network : Subsystem
      mask help: Swap bytes of an uint32 value from host byte-order to network byte-order (big-endian).
      mask DialogControl DescGroupVar Prompt: Swap Uint32 Host To Network
      mask Display: disp('hton (uint32)');

== system AVE_Library/Essential/Positive Angle ==
  in : Inport  OutDataTypeStr=double  Unit=rad
  MATLAB Function : MATLAB Function  TreatAsAtomicUnit=on
  out : Outport  OutDataTypeStr=double  Unit=rad  VectorParamsAs1DForOutWhenUnconnected=off
  wires:
  in/1 -> MATLAB Function/1(u)
  MATLAB Function/1(y) -> out/1

== system AVE_Library/Essential/Replace NaN ==
  in : Inport  OutDataTypeStr=double
  MATLAB Function : MATLAB Function  TreatAsAtomicUnit=on
  out : Outport  OutDataTypeStr=double
  wires:
  in/1 -> MATLAB Function/1(u)
  MATLAB Function/1(y) -> out/1

== system AVE_Library/Essential/Replace Nonfinite ==
  in : Inport
  MATLAB Function : MATLAB Function  TreatAsAtomicUnit=on
  out : Outport
  wires:
  in/1 -> MATLAB Function/1(u)
  MATLAB Function/1(y) -> out/1

== system AVE_Library/Essential/SHA256 ==
  bytes : Inport  OutDataTypeStr=uint8
  numBytes : Inport  Port=2  PortDimensions=1
  SHA256 : MATLAB Function  TreatAsAtomicUnit=on
  hash : Outport  OutDataTypeStr=uint8  PortDimensions=32
  wires:
  bytes/1 -> SHA256/1(bytes)
  numBytes/1 -> SHA256/2(numBytes)
  SHA256/1(hash) -> hash/1

== system AVE_Library/Essential/Safe Normalization ==
  in : Inport  OutDataTypeStr=double
  AND : Logic  AllPortsSameDT=off  OutDataTypeStr=boolean
  AND1 : Logic  Inputs=1  AllPortsSameDT=off  OutDataTypeStr=boolean
  Assignment : Assignment  DiagnosticForDimensions=Warning  IndexOptions=Index vector (dialog)  Indices=1  OutputSizes=1
  Compare To Constant : simulink/Logic and Bit Operations/Compare To Constant  relop=>  const=1e-12  OutDataTypeStr=boolean
  Gain : Gain  Gain=0
  Is Finite : $bdroot/Essential/Is Finite
  One : Constant
  Product1 : Product  Inputs=*/
  Replace NaN : $bdroot/Essential/Replace NaN  value=0.0
  Sqrt : Sqrt
  Square : Math  Operator=square
  Sum of Elements : Sum  Inputs=+
  Switch : Switch  Criteria=u2 ~= 0  Threshold=1e-12  SaturateOnIntegerOverflow=off  InputSameDT=off
  out : Outport  OutDataTypeStr=double
  wires:
  Square/1 -> Sum of Elements/1
  Product1/1 -> Switch/1
  Sqrt/1 -> Compare To Constant/1, Product1/2
  in/1 -> Square/1, Gain/1, Is Finite/1, Product1/1
  Sum of Elements/1 -> Sqrt/1
  One/1 -> Assignment/2
  Switch/1 -> out/1
  Assignment/1 -> Switch/3
  Compare To Constant/1 -> AND/2
  AND/1 -> Switch/2
  AND1/1 -> AND/1
  Gain/1 -> Replace NaN/1
  Replace NaN/1 -> Assignment/1
  Is Finite/1 -> AND1/1

== system AVE_Library/Essential/Signal Logics ==
  Hold Timeout : Subsystem
      mask help: Hold timeout at tfTimeout inport for at least timeToHold.
      mask DialogControl DescGroupVar Prompt: Hold Timeout
      mask Display: disp('Hold Timeout');
  Index Of Latest Trigger : Subsystem
      mask help: Get the zero-based index of the element in the input vector that is enabled (rising edge).
      mask DialogControl DescGroupVar Prompt: Index Of Latest Trigger
  Index To Enable Vector : Subsystem  mask{outputSize=1}
      mask prompts: outputSize "Output vector size (0 ... 255):"
      mask help: Create a boolean vector of "false" values, where one value (idx) is true. idx indicates a zero-based index.
      mask DialogControl DescGroupVar Prompt: Index To Enable Vector
  Push Buttons To Toggle Switches : Subsystem
      mask help:
      | Convert push button events (rising edge events) to toggle switches. If a push button input is changed from false to true, then the corresponding boolean switch output is toggled, e.g. inverted. As long as the reset input is true, all internal toggle states are reset (overwritten) to false.<br><br>
      | <br><table border="1" align="center" width="100%"><tr><th>Input</th></tr></table><br><br>
      | <b>pushButtons</b><br>
      | Boolean push button events where true means pushed and false means released. This can be a multi-dimensional signal.<br><br>
      | <b>reset</b><br>
      | If the reset input is true, the internal toggle states for all buttons is reset to false.<br><br>
      | <br><table border="1" align="center" width="100%"><tr><th>Output</th></tr></table><br><br>
      | <b>toggleSwitches</b><br>
      | The state of toggle switches where true means enabled and false means disabled. The dimension is equal to that of the pushButtons input.
      mask DialogControl DescGroupVar Prompt: Push Buttons To Toggle Switches
      mask Display: disp('Push Buttons\nTo\nToggle Switches');
  Resetable Index Of Latest Trigger : Subsystem
      mask help: Get the zero-based index of the element in the input vector that is enabled (rising edge). If the reset input is enabled, then the internal value is reset to the specified resetValue.
      mask DialogControl DescGroupVar Prompt: Resetable Index Of Latest Trigger
  Resetable Toggle Value Up : Subsystem  mask{maxValue=1}
      mask prompts: maxValue "Maximum value:"
      mask help: Toggle from zero to a maximum value. The value is incremented each time the triggerUp has a rising edge. If reset is true, then the internal value is reset (zero).
      mask DialogControl DescGroupVar Prompt: Resetable Toggle Value Up
  Time To Latest Event : Subsystem
      mask help:
      | Calculate the time to the latest event. The initial output is Inf. As long as the event input is true, the output is zero.<br><br>
      | <br><table border="1" align="center" width="100%"><tr><th>Input</th></tr></table><br><br>
      | <b>event</b><br>
      | A boolean value that is true if the event has occurred.<br><br>
      | <b>steadyClock</b><br>
      | A time source that represents a monotonically increasing time in seconds.<br><br>
      | <br><table border="1" align="center" width="100%"><tr><th>Output</th></tr></table><br><br>
      | <b>timeToLatestEvent</b><br>
      | Time to the latest event. The initial output is Inf. If event is TRUE, then this output is zero.
      mask DialogControl DescGroupVar Prompt: Time To Latest Event
      mask Display: disp('Time\nTo\nLatest Event');
  Toggle Value Up : Subsystem  mask{maxValue=1}
      mask prompts: maxValue "Maximum value:"
      mask help: Toggle from zero to a maximum value. The value is incremented each time the triggerUp has a rising edge.
      mask DialogControl DescGroupVar Prompt: Toggle Value Up
  Toggle Value Up Down : Subsystem  mask{maxValue=1}
      mask prompts: maxValue "Maximum value:"
      mask help: Toggle between zero and maximum value. The value is incremented or decremented each time the respective trigger has a rising edge.
      mask DialogControl DescGroupVar Prompt: Toggle Value Up Down
  Trigger Generator : Subsystem  mask{SampleTime=-1}
      mask prompts: SampleTime "Sample time (-1 for inherited):"
      mask help:
      | Generate a periodic trigger signal. The trigger is high every time the trigger sampletime expires. The internal counter can be reset by the external reset input.<br><br>
      | <br><table border="1" align="center" width="100%"><tr><th>Input</th></tr></table><br><br>
      | <b>triggerPeriod</b><br>
      | The trigger period in seconds.<br><br>
      | <b>reset</b><br>
      | If the reset input is high, the internal counter is reset and the trigger output is high.<br><br>
      | <br><table border="1" align="center" width="100%"><tr><th>Output</th></tr></table><br><br>
      | <b>trigger</b><br>
      | A periodic pulse signal, where the time interval of the pulses is defined by triggerPeriod.
      mask DialogControl DescGroupVar Prompt: Trigger Generator
      mask Display: disp('Trigger\nGenerator');

== system AVE_Library/Essential/Smoothstep ==
  edge0 : Inport  OutDataTypeStr=double  PortDimensions=1
  edge1 : Inport  Port=2  OutDataTypeStr=double  PortDimensions=1
  in : Inport  Port=3  OutDataTypeStr=double  PortDimensions=1
  MATLAB Function : MATLAB Function  TreatAsAtomicUnit=on
  out : Outport  OutDataTypeStr=double  PortDimensions=1  VectorParamsAs1DForOutWhenUnconnected=off
  wires:
  edge0/1 -> MATLAB Function/1(edge0)
  edge1/1 -> MATLAB Function/2(edge1)
  MATLAB Function/1(y) -> out/1
  in/1 -> MATLAB Function/3(x)

== system AVE_Library/Essential/Symmetrical Angle ==
  in : Inport  OutDataTypeStr=double  Unit=rad
  MATLAB Function1 : MATLAB Function  TreatAsAtomicUnit=on
  out : Outport  OutDataTypeStr=double  Unit=rad  VectorParamsAs1DForOutWhenUnconnected=off
  wires:
  MATLAB Function1/1(y) -> out/1
  in/1 -> MATLAB Function1/1(u)
